simulink model "PVAndBatteryIntegratedPlantForBlackStart"  (R2025b)
settings: Solver=FixedStepAuto  StartTime=0.0  StopTime=tsim  FixedStep=1e-6  RelTol=1e-9  AbsTol=1e-7
InitFcn:
  | %% Black Start Sequence
  | t0 = 0; % Battery IBR initial time
  | t1 = 0.15; % PV IBR initial time
  | t2 = 0.5; % Two IBR sync time
  | t3 = 0.8; % Additional motor load connect
  | t4 = 1.1; % Grid reconnection
  | tsim = 1.5; % Total simulation time
  | 
  | %% initialize
  | Vdc = 400;
  | Vnom = 100;
  | Prated = 10000;
  | Qrated = 0;
  | Srated = sqrt(Prated^2+Qrated^2);
  | wnom = 2*pi*60;
  | fnom = 60;
  | Vminpu = 0.95;
  | 
  | kv = Vnom;
  | ki = 3*Vnom/Srated;
  | 
  | dwmax = 0.5*2*pi;
  | trisemax = 0.1;
  | 
  | C = 1/sqrt(2)/Vminpu^2/dwmax;
  | L = 1/C/wnom^2;
  | tau = C/kv/ki;
  | epsilon = sqrt(L/C);
  | ksy = 3/2/trisemax;
  | 
  | V_voc_1 = 0;
  | V_voc_2 = 0;
  | 
  | % filter
  | Rf = 0.05;
  | Lf = 500e-6;
  | % pwm
  | fsw = 10e3;
  | % simulation
  | Ts = 1e-6;
  | 
  | % load
  | Rl = 3*Vnom^2/Prated;
  | Rl1 = Rl;
  | Rl2 = 2*Rl;
  | Rl3 = 20*Rl;
  | % grid
  | Rg = 0.05;
  | Lg = 50e-6;
  | 
  | % DCDC converter
  | Kp_V = 1;
  | Ki_V = 0.02;
  | Imax = 110;
  | Kp_I = 0.0001;
  | Ki_I = 1;
  | Vcmax = 1;
undefined symbols (not defined in the file): alpha, C_voc, Diode_class, Half_BridgeConverter_class, L_voc, Ll, Mosfet_class, PWMGenerator_DC_DC__class, R_voc, Three_PhaseBreaker_class, Three_PhaseSource_class, Three_PhaseTransformer_2_class, Three_PhaseV_IMeasuremen_class
libraries: nesl_utility x69, ee_lib x49, fl_lib x36, mcbeeMathTransformLib x9, simulink x6, spsParallelRLCBranchLib x3, eePwmGeneratorTwoLevel x2, spsControlledCurrentSourceLib x2, elec_conv_HighZElecRef x2, slpidlib x2, spsSecondOrderFilterLib x1, spsCurrentMeasurementLib x1
(part 2 of 4)

== system PVAndBatteryIntegratedPlantForBlackStart/prim4 ==
  Current and Voltage Sensor (Three-Phase) : ee_lib/Sensors & Transducers/Current and Voltage Sensor (Three-Phase)  vMeasurementType=2  outputUnit=2  SRated=100000000 V*A  VRated=500000 V  I_specify=off  I_priority=None  I=[ 0 0 0 ] A  I_nominal_specify=off  I_nominal_value=1  I_nominal_unit=A  V_specify=off  V_priority=None  V=[ 0 0 0 ] V  V_nominal_specify=off  V_nominal_value=1  V_nominal_unit=V
      settings: InternalSimscapePortConfiguration="{\"Bottom\":[],\"Left\":[{\"id\":\"a1\",\"label\":\"a1\",\"type\":\"foundation.electrical.electrical\"},{\"id\":\"b1\",\"label\":\"b1\",\"type\":\"foundation.electrical.electrical\"},{\"id\":\"c1\",\"label\":\"c1\",\"type\":\"foundation.electrical.electrical\"}],\"Right\":[{\"id\":\"V_output\",\"label\":\"V\",\"type\":\"output\"},{\"id\":\"I_output\",\"label\":\"I\",\"type\":\"output\"},{\"id\":\"a2\",\"label\":\"a2\",\"type\":\"foundation.electrical.electrical\"},{\"id\":\"b2\",\"label\":\"b2\",\"type\":\"foundation.electrical.electrical\"},{\"id\":\"c2\",\"label\":\"c2\",\"type\":\"foundation.electrical.electrical\"}],\"Top\":[]}"
  Igain : Gain  Gain=Three_PhaseV_IMeasuremen_class('phase-to-ground','yes','off','off','off',100000000,500000).objParamMappingDerived.NewDerivedParam.IG
  PS-Simulink Converter : nesl_utility/PS-Simulink Converter  PhysicalDomain=network_engine_domain  SubClassName=ps_output  LeftPortType=input  RightPortType=output  PseudoPeriodic=off  Frequencies=[]  VectorFormat=1-D array  Unit=1  AffineConversion=off
  PS-Simulink Converter1 : nesl_utility/PS-Simulink Converter  PhysicalDomain=network_engine_domain  SubClassName=ps_output  LeftPortType=input  RightPortType=output  PseudoPeriodic=off  Frequencies=[]  VectorFormat=1-D array  Unit=1  AffineConversion=off
  Vgain : Gain  Gain=Three_PhaseV_IMeasuremen_class('phase-to-ground','yes','off','off','off',100000000,500000).objParamMappingDerived.NewDerivedParam.VG
  A : PMIOPort  Side=Left
  B : PMIOPort  Port=2  Side=Left
  C : PMIOPort  Port=3  Side=Left
  a : PMIOPort  Port=4  Side=Right
  b : PMIOPort  Port=5  Side=Right
  c : PMIOPort  Port=6  Side=Right
  Vabc : Outport  VectorParamsAs1DForOutWhenUnconnected=off
  Iabc : Outport  Port=2  VectorParamsAs1DForOutWhenUnconnected=off
  wires:
  Igain/1 -> Iabc/1
  Vgain/1 -> Vabc/1
  PS-Simulink Converter1/1 -> Igain/1
  PS-Simulink Converter/1 -> Vgain/1
  connections:
  Current and Voltage Sensor (Three-Phase)/RConn1 -- PS-Simulink Converter/LConn1
  Current and Voltage Sensor (Three-Phase)/RConn2 -- PS-Simulink Converter1/LConn1
  Current and Voltage Sensor (Three-Phase)/RConn5 -- c/RConn1
  Current and Voltage Sensor (Three-Phase)/RConn4 -- b/RConn1
  Current and Voltage Sensor (Three-Phase)/RConn3 -- a/RConn1
  Current and Voltage Sensor (Three-Phase)/LConn3 -- C/RConn1
  Current and Voltage Sensor (Three-Phase)/LConn1 -- A/RConn1
  Current and Voltage Sensor (Three-Phase)/LConn2 -- B/RConn1

== system PVAndBatteryIntegratedPlantForBlackStart/Battery Inverter/DC Voltage Source ==
  DC Voltage Source : fl_lib/Electrical/Electrical Sources/DC Voltage Source  v0=Vdc V
  - : PMIOPort  Side=Left
  + : PMIOPort  Port=2  Side=Right
  connections:
  DC Voltage Source/RConn1 -- -/RConn1
  DC Voltage Source/LConn1 -- +/RConn1

== system PVAndBatteryIntegratedPlantForBlackStart/Battery Inverter/Feedback ==
  In2 : Inport
  Enable : EnablePort
  Ifb : Outport
  wires:
  In2/1 -> Ifb/1

== system PVAndBatteryIntegratedPlantForBlackStart/Battery Inverter/Inverter ==
  g : Inport
  Constant : Constant  Value=0
  Demux : Demux  Outputs=6
  Half-Bridge Converter : Subsystem
  Half-Bridge Converter1 : Subsystem
      settings: OpenFcn=elec.conv.unmask(gcb);
  Half-Bridge Converter2 : Subsystem
      settings: OpenFcn=elec.conv.unmask(gcb);
  Mux : Mux  Inputs=2
  Mux1 : Mux  Inputs=2
  Mux2 : Mux  Inputs=2
  Vdc+ : PMIOPort  Side=Left
  Vdc- : PMIOPort  Port=2  Side=Left
  Va : PMIOPort  Port=3  Side=Right
  Vb : PMIOPort  Port=4  Side=Right
  Vc : PMIOPort  Port=5  Side=Right
  wires:
  g/1 -> Demux/1
  Constant/1 -> Half-Bridge Converter2/2(BL), Half-Bridge Converter1/2(BL), Half-Bridge Converter/2(BL)
  Demux/1 -> Mux/1
  Demux/2 -> Mux/2
  Demux/4 -> Mux1/2
  Demux/3 -> Mux1/1
  Demux/5 -> Mux2/1
  Demux/6 -> Mux2/2
  Mux/1 -> Half-Bridge Converter/1(" g ")
  Mux1/1 -> Half-Bridge Converter1/1(" g ")
  Mux2/1 -> Half-Bridge Converter2/1(" g ")
  connections:
  Half-Bridge Converter/RConn1 -- Half-Bridge Converter2/RConn1 -- Half-Bridge Converter1/RConn1 -- Vdc+/RConn1
  Vdc-/RConn1 -- Half-Bridge Converter2/RConn2 -- Half-Bridge Converter1/RConn2 -- Half-Bridge Converter/RConn2
  Half-Bridge Converter1/LConn1 -- Vb/RConn1
  Vc/RConn1 -- Half-Bridge Converter2/LConn1
  Va/RConn1 -- Half-Bridge Converter/LConn1

== system PVAndBatteryIntegratedPlantForBlackStart/Battery Inverter/L1 ==
  Three_PhaseSeriesRLCBran : ee_lib/Passive/RLC Assemblies/RLC (Three-Phase)  port_option=ee.enum.threePhasePort.expanded  component_structure=4  R=Rf Ohm  L=Lf H  C=Inf F  R_parasitic=1e-6 Ohm  G_parasitic=1e-6 1/Ohm  IL_specify=on  IL_priority=High  IL=[0, 0, 0] A  IL_nominal_specify=off  IL_nominal_value=1  IL_nominal_unit=A  VC_specify=on  VC_priority=High  VC=[0, 0, 0] V  VC_nominal_specify=off  VC_nominal_value=1  VC_nominal_unit=V
      settings: InternalSimscapePortConfiguration="{\"Bottom\":[],\"Left\":[{\"id\":\"a1\",\"label\":\"a1\",\"type\":\"foundation.electrical.electrical\"},{\"id\":\"b1\",\"label\":\"b1\",\"type\":\"foundation.electrical.electrical\"},{\"id\":\"c1\",\"label\":\"c1\",\"type\":\"foundation.electrical.electrical\"}],\"Right\":[{\"id\":\"a2\",\"label\":\"a2\",\"type\":\"foundation.electrical.electrical\"},{\"id\":\"b2\",\"label\":\"b2\",\"type\":\"foundation.electrical.electrical\"},{\"id\":\"c2\",\"label\":\"c2\",\"type\":\"foundation.electrical.electrical\"}],\"Top\":[]}"
  A : PMIOPort  Side=Left
  B : PMIOPort  Port=2  Side=Left
  C : PMIOPort  Port=3  Side=Left
  a : PMIOPort  Port=4  Side=Right
  b : PMIOPort  Port=5  Side=Right
  c : PMIOPort  Port=6  Side=Right
  connections:
  Three_PhaseSeriesRLCBran/RConn3 -- c/RConn1
  Three_PhaseSeriesRLCBran/RConn2 -- b/RConn1
  Three_PhaseSeriesRLCBran/RConn1 -- a/RConn1
  C/RConn1 -- Three_PhaseSeriesRLCBran/LConn3
  B/RConn1 -- Three_PhaseSeriesRLCBran/LConn2
  A/RConn1 -- Three_PhaseSeriesRLCBran/LConn1

== system PVAndBatteryIntegratedPlantForBlackStart/Battery Inverter/Three-Phase Breaker ==
  com : Inport
  Add : Sum
  Circuit Breaker : ee_lib/Switches & Breakers/Circuit Breaker (Three-Phase)  R_closed=0.001 Ohm  G_open=Three_PhaseBreaker_class('open',1000000,Inf,[0.0166666666666667 0.0833333333333333],'on').objParamMappingDerived.NewDerivedParam.G_open 1/Ohm  threshold=0.5 V  breaker_behavior=ee.enum.switches.breakerBehavior.zeroCrossingEnable
      settings: InternalSimscapePortConfiguration="{\"Bottom\":[],\"Left\":[{\"id\":\"vT\",\"label\":\"vT\",\"type\":\"input\"},{\"id\":\"a1\",\"label\":\"a1\",\"type\":\"foundation.electrical.electrical\"},{\"id\":\"b1\",\"label\":\"b1\",\"type\":\"foundation.electrical.electrical\"},{\"id\":\"c1\",\"label\":\"c1\",\"type\":\"foundation.electrical.electrical\"}],\"Right\":[{\"id\":\"a2\",\"label\":\"a2\",\"type\":\"foundation.electrical.electrical\"},{\"id\":\"b2\",\"label\":\"b2\",\"type\":\"foundation.electrical.electrical\"},{\"id\":\"c2\",\"label\":\"c2\",\"type\":\"foundation.electrical.electrical\"}],\"Top\":[]}"
  Data Type Conversion : DataTypeConversion  OutDataTypeStr=double  SaturateOnIntegerOverflow=off  RndMeth=Floor
  NOT : Logic  Operator=NOT  IconShape=distinctive  AllPortsSameDT=off  OutDataTypeStr=boolean
  Simulink-PS Converter : nesl_utility/Simulink-PS Converter  PhysicalDomain=network_engine_domain  SubClassName=ps_input  LeftPortType=input  RightPortType=output  PseudoPeriodic=off  Frequencies=[]  NoiseDistribution=none  NoiseParameters=[]  Unit=1  AffineConversion=off  FilteringAndDerivatives=provide  SimscapeFilterOrder=1  InputFilterTimeConstant=0.001  UdotUserProvided=0
  Step : Step  Time=1e-6  Before=Three_PhaseBreaker_class('open',1000000,Inf,[0.0166666666666667 0.0833333333333333],'on').objParamMappingDerived.NewDerivedParam.StepInitialValue  After=0  SampleTime=0
  A : PMIOPort  Side=Left
  B : PMIOPort  Port=2  Side=Left
  C : PMIOPort  Port=3  Side=Left
  a : PMIOPort  Port=4  Side=Right
  b : PMIOPort  Port=5  Side=Right
  c : PMIOPort  Port=6  Side=Right
  wires:
  com/1 -> Add/1
  Add/1 -> NOT/1
  Step/1 -> Add/2
  Data Type Conversion/1 -> Simulink-PS Converter/1
  NOT/1 -> Data Type Conversion/1
  connections:
  Circuit Breaker/LConn1 -- Simulink-PS Converter/RConn1
  c/RConn1 -- Circuit Breaker/RConn3
  b/RConn1 -- Circuit Breaker/RConn2
  a/RConn1 -- Circuit Breaker/RConn1
  Circuit Breaker/LConn4 -- C/RConn1
  Circuit Breaker/LConn3 -- B/RConn1
  Circuit Breaker/LConn2 -- A/RConn1

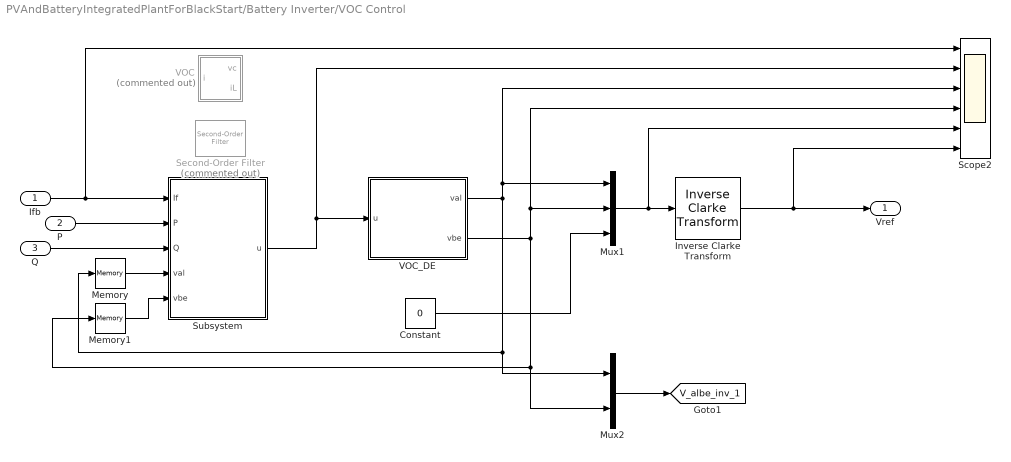
== system PVAndBatteryIntegratedPlantForBlackStart/Battery Inverter/VOC Control ==
  Ifb : Inport
  P : Inport  Port=2
  Q : Inport  Port=3
  Constant : Constant  Value=0
  Inverse Clarke Transform : mcbeeMathTransformLib/Inverse Clarke Transform  PowerInvariant=off  UseWithEmbedded=off  PhaseInput=Two inputs
      settings: LibrarySourceBlock=|
      | ee_sl_lib/Mathematical
      | Transforms/Inverse
      | Clarke Transform
  Memory : Memory
  Memory1 : Memory
  Mux1 : Mux  Inputs=3
  Mux2 : Mux  Inputs=2
  Scope2 : Scope  NumInputPorts=6
      settings: ActiveDisplayYMinimum=-957.42377  ActiveDisplayYMaximum=1099.35573
  Second-Order Filter : spsSecondOrderFilterLib/Second-Order Filter  Commented=on  FilterType=Lowpass  Fo=fnom*10  Zeta=0.707  Ts=0  Initialize=on  Vac_Init="[0,  0,  60]"  Vdc_Init=0  PlotResponse=off  FreqRange=[0, 500, 1]
      settings: LibrarySourceBlock=|
      | sps_lib/Control/Filters/Second-Order
      | Filter
  Subsystem : Subsystem
  VOC : Subsystem  Commented=on
  VOC_DE : Subsystem
  Vref : Outport
  tag scope: V_albe_inv_1=global
  wires:
  Memory1/1 -> Subsystem/5(vbe)
  Memory/1 -> Subsystem/4(val)
  Mux1/1 -> Scope2/5, Inverse Clarke Transform/1
  Ifb/1 -> Subsystem/1(If), Scope2/1
  Inverse Clarke Transform/1 -> Vref/1, Scope2/6
  VOC_DE/1(val) -> Mux2/1, Memory/1, Scope2/3, Mux1/1
  VOC_DE/2(vbe) -> Scope2/4, Mux1/2, Mux2/2, Memory1/1
  Constant/1 -> Mux1/3
  Subsystem/1(u) -> Scope2/2, VOC_DE/1(u)
  P/1 -> Subsystem/2(P)
  Q/1 -> Subsystem/3(Q)
  Mux2/1 -> [V_albe_inv_1]

== system PVAndBatteryIntegratedPlantForBlackStart/Battery Inverter/inv ==
  Current and Voltage Sensor (Three-Phase) : ee_lib/Sensors & Transducers/Current and Voltage Sensor (Three-Phase)  vMeasurementType=2  outputUnit=2  SRated=100000000 V*A  VRated=500000 V  I_specify=off  I_priority=None  I=[ 0 0 0 ] A  I_nominal_specify=off  I_nominal_value=1  I_nominal_unit=A  V_specify=off  V_priority=None  V=[ 0 0 0 ] V  V_nominal_specify=off  V_nominal_value=1  V_nominal_unit=V
      settings: InternalSimscapePortConfiguration="{\"Bottom\":[],\"Left\":[{\"id\":\"a1\",\"label\":\"a1\",\"type\":\"foundation.electrical.electrical\"},{\"id\":\"b1\",\"label\":\"b1\",\"type\":\"foundation.electrical.electrical\"},{\"id\":\"c1\",\"label\":\"c1\",\"type\":\"foundation.electrical.electrical\"}],\"Right\":[{\"id\":\"V_output\",\"label\":\"V\",\"type\":\"output\"},{\"id\":\"I_output\",\"label\":\"I\",\"type\":\"output\"},{\"id\":\"a2\",\"label\":\"a2\",\"type\":\"foundation.electrical.electrical\"},{\"id\":\"b2\",\"label\":\"b2\",\"type\":\"foundation.electrical.electrical\"},{\"id\":\"c2\",\"label\":\"c2\",\"type\":\"foundation.electrical.electrical\"}],\"Top\":[]}"
  Igain : Gain  Gain=Three_PhaseV_IMeasuremen_class('phase-to-ground','yes','off','off','off',100000000,500000).objParamMappingDerived.NewDerivedParam.IG
  PS-Simulink Converter : nesl_utility/PS-Simulink Converter  PhysicalDomain=network_engine_domain  SubClassName=ps_output  LeftPortType=input  RightPortType=output  PseudoPeriodic=off  Frequencies=[]  VectorFormat=1-D array  Unit=1  AffineConversion=off
  PS-Simulink Converter1 : nesl_utility/PS-Simulink Converter  PhysicalDomain=network_engine_domain  SubClassName=ps_output  LeftPortType=input  RightPortType=output  PseudoPeriodic=off  Frequencies=[]  VectorFormat=1-D array  Unit=1  AffineConversion=off
  Vgain : Gain  Gain=Three_PhaseV_IMeasuremen_class('phase-to-ground','yes','off','off','off',100000000,500000).objParamMappingDerived.NewDerivedParam.VG
  A : PMIOPort  Side=Left
  B : PMIOPort  Port=2  Side=Left
  C : PMIOPort  Port=3  Side=Left
  a : PMIOPort  Port=4  Side=Right
  b : PMIOPort  Port=5  Side=Right
  c : PMIOPort  Port=6  Side=Right
  Vabc : Outport  VectorParamsAs1DForOutWhenUnconnected=off
  Iabc : Outport  Port=2  VectorParamsAs1DForOutWhenUnconnected=off
  wires:
  Igain/1 -> Iabc/1
  Vgain/1 -> Vabc/1
  PS-Simulink Converter1/1 -> Igain/1
  PS-Simulink Converter/1 -> Vgain/1
  connections:
  Current and Voltage Sensor (Three-Phase)/RConn1 -- PS-Simulink Converter/LConn1
  Current and Voltage Sensor (Three-Phase)/RConn2 -- PS-Simulink Converter1/LConn1
  Current and Voltage Sensor (Three-Phase)/RConn5 -- c/RConn1
  Current and Voltage Sensor (Three-Phase)/RConn4 -- b/RConn1
  Current and Voltage Sensor (Three-Phase)/RConn3 -- a/RConn1
  Current and Voltage Sensor (Three-Phase)/LConn3 -- C/RConn1
  Current and Voltage Sensor (Three-Phase)/LConn1 -- A/RConn1
  Current and Voltage Sensor (Three-Phase)/LConn2 -- B/RConn1

== system PVAndBatteryIntegratedPlantForBlackStart/Battery Inverter/inv1 ==
  Current and Voltage Sensor (Three-Phase) : ee_lib/Sensors & Transducers/Current and Voltage Sensor (Three-Phase)  vMeasurementType=2  outputUnit=2  SRated=100000000 V*A  VRated=500000 V  I_specify=off  I_priority=None  I=[ 0 0 0 ] A  I_nominal_specify=off  I_nominal_value=1  I_nominal_unit=A  V_specify=off  V_priority=None  V=[ 0 0 0 ] V  V_nominal_specify=off  V_nominal_value=1  V_nominal_unit=V
      settings: InternalSimscapePortConfiguration="{\"Bottom\":[],\"Left\":[{\"id\":\"a1\",\"label\":\"a1\",\"type\":\"foundation.electrical.electrical\"},{\"id\":\"b1\",\"label\":\"b1\",\"type\":\"foundation.electrical.electrical\"},{\"id\":\"c1\",\"label\":\"c1\",\"type\":\"foundation.electrical.electrical\"}],\"Right\":[{\"id\":\"V_output\",\"label\":\"V\",\"type\":\"output\"},{\"id\":\"I_output\",\"label\":\"I\",\"type\":\"output\"},{\"id\":\"a2\",\"label\":\"a2\",\"type\":\"foundation.electrical.electrical\"},{\"id\":\"b2\",\"label\":\"b2\",\"type\":\"foundation.electrical.electrical\"},{\"id\":\"c2\",\"label\":\"c2\",\"type\":\"foundation.electrical.electrical\"}],\"Top\":[]}"
  Igain : Gain  Gain=Three_PhaseV_IMeasuremen_class('phase-to-ground','yes','off','off','off',100000000,500000).objParamMappingDerived.NewDerivedParam.IG
  PS-Simulink Converter : nesl_utility/PS-Simulink Converter  PhysicalDomain=network_engine_domain  SubClassName=ps_output  LeftPortType=input  RightPortType=output  PseudoPeriodic=off  Frequencies=[]  VectorFormat=1-D array  Unit=1  AffineConversion=off
  PS-Simulink Converter1 : nesl_utility/PS-Simulink Converter  PhysicalDomain=network_engine_domain  SubClassName=ps_output  LeftPortType=input  RightPortType=output  PseudoPeriodic=off  Frequencies=[]  VectorFormat=1-D array  Unit=1  AffineConversion=off
  Vgain : Gain  Gain=Three_PhaseV_IMeasuremen_class('phase-to-ground','yes','off','off','off',100000000,500000).objParamMappingDerived.NewDerivedParam.VG
  A : PMIOPort  Side=Left
  B : PMIOPort  Port=2  Side=Left
  C : PMIOPort  Port=3  Side=Left
  a : PMIOPort  Port=4  Side=Right
  b : PMIOPort  Port=5  Side=Right
  c : PMIOPort  Port=6  Side=Right
  Vabc : Outport  VectorParamsAs1DForOutWhenUnconnected=off
  Iabc : Outport  Port=2  VectorParamsAs1DForOutWhenUnconnected=off
  wires:
  Igain/1 -> Iabc/1
  Vgain/1 -> Vabc/1
  PS-Simulink Converter1/1 -> Igain/1
  PS-Simulink Converter/1 -> Vgain/1
  connections:
  Current and Voltage Sensor (Three-Phase)/RConn1 -- PS-Simulink Converter/LConn1
  Current and Voltage Sensor (Three-Phase)/RConn2 -- PS-Simulink Converter1/LConn1
  Current and Voltage Sensor (Three-Phase)/RConn5 -- c/RConn1
  Current and Voltage Sensor (Three-Phase)/RConn4 -- b/RConn1
  Current and Voltage Sensor (Three-Phase)/RConn3 -- a/RConn1
  Current and Voltage Sensor (Three-Phase)/LConn3 -- C/RConn1
  Current and Voltage Sensor (Three-Phase)/LConn1 -- A/RConn1
  Current and Voltage Sensor (Three-Phase)/LConn2 -- B/RConn1

== system PVAndBatteryIntegratedPlantForBlackStart/Linear Load 2/Three-Phase Series RLC Branch1 ==
  Three_PhaseSeriesRLCBran : ee_lib/Passive/RLC Assemblies/RLC (Three-Phase)  port_option=ee.enum.threePhasePort.expanded  component_structure=1  R=Rl2 Ohm  L=Ll H  C=1e-06 F  R_parasitic=1e-6 Ohm  G_parasitic=1e-6 1/Ohm  IL_specify=on  IL_priority=High  IL=[0, 0, 0] A  IL_nominal_specify=off  IL_nominal_value=1  IL_nominal_unit=A  VC_specify=on  VC_priority=High  VC=[0, 0, 0] V  VC_nominal_specify=off  VC_nominal_value=1  VC_nominal_unit=V
      settings: InternalSimscapePortConfiguration="{\"Bottom\":[],\"Left\":[{\"id\":\"a1\",\"label\":\"a1\",\"type\":\"foundation.electrical.electrical\"},{\"id\":\"b1\",\"label\":\"b1\",\"type\":\"foundation.electrical.electrical\"},{\"id\":\"c1\",\"label\":\"c1\",\"type\":\"foundation.electrical.electrical\"}],\"Right\":[{\"id\":\"a2\",\"label\":\"a2\",\"type\":\"foundation.electrical.electrical\"},{\"id\":\"b2\",\"label\":\"b2\",\"type\":\"foundation.electrical.electrical\"},{\"id\":\"c2\",\"label\":\"c2\",\"type\":\"foundation.electrical.electrical\"}],\"Top\":[]}"
  A : PMIOPort  Side=Left
  B : PMIOPort  Port=2  Side=Left
  C : PMIOPort  Port=3  Side=Left
  a : PMIOPort  Port=4  Side=Right
  b : PMIOPort  Port=5  Side=Right
  c : PMIOPort  Port=6  Side=Right
  connections:
  Three_PhaseSeriesRLCBran/RConn3 -- c/RConn1
  Three_PhaseSeriesRLCBran/RConn2 -- b/RConn1
  Three_PhaseSeriesRLCBran/RConn1 -- a/RConn1
  C/RConn1 -- Three_PhaseSeriesRLCBran/LConn3
  B/RConn1 -- Three_PhaseSeriesRLCBran/LConn2
  A/RConn1 -- Three_PhaseSeriesRLCBran/LConn1

== system PVAndBatteryIntegratedPlantForBlackStart/Linear load 1/Three-Phase Series RLC Branch ==
  Three_PhaseSeriesRLCBran : ee_lib/Passive/RLC Assemblies/RLC (Three-Phase)  port_option=ee.enum.threePhasePort.expanded  component_structure=1  R=Rl1 Ohm  L=Ll H  C=1e-06 F  R_parasitic=1e-6 Ohm  G_parasitic=1e-6 1/Ohm  IL_specify=on  IL_priority=High  IL=[0, 0, 0] A  IL_nominal_specify=off  IL_nominal_value=1  IL_nominal_unit=A  VC_specify=on  VC_priority=High  VC=[0, 0, 0] V  VC_nominal_specify=off  VC_nominal_value=1  VC_nominal_unit=V
      settings: InternalSimscapePortConfiguration="{\"Bottom\":[],\"Left\":[{\"id\":\"a1\",\"label\":\"a1\",\"type\":\"foundation.electrical.electrical\"},{\"id\":\"b1\",\"label\":\"b1\",\"type\":\"foundation.electrical.electrical\"},{\"id\":\"c1\",\"label\":\"c1\",\"type\":\"foundation.electrical.electrical\"}],\"Right\":[{\"id\":\"a2\",\"label\":\"a2\",\"type\":\"foundation.electrical.electrical\"},{\"id\":\"b2\",\"label\":\"b2\",\"type\":\"foundation.electrical.electrical\"},{\"id\":\"c2\",\"label\":\"c2\",\"type\":\"foundation.electrical.electrical\"}],\"Top\":[]}"
  A : PMIOPort  Side=Left
  B : PMIOPort  Port=2  Side=Left
  C : PMIOPort  Port=3  Side=Left
  a : PMIOPort  Port=4  Side=Right
  b : PMIOPort  Port=5  Side=Right
  c : PMIOPort  Port=6  Side=Right
  connections:
  Three_PhaseSeriesRLCBran/RConn3 -- c/RConn1
  Three_PhaseSeriesRLCBran/RConn2 -- b/RConn1
  Three_PhaseSeriesRLCBran/RConn1 -- a/RConn1
  C/RConn1 -- Three_PhaseSeriesRLCBran/LConn3
  B/RConn1 -- Three_PhaseSeriesRLCBran/LConn2
  A/RConn1 -- Three_PhaseSeriesRLCBran/LConn1

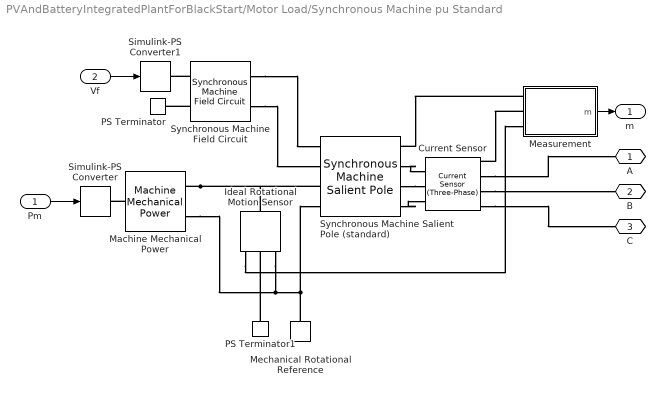
== system PVAndBatteryIntegratedPlantForBlackStart/Motor Load/Synchronous Machine pu Standard ==
  Pm : Inport
  Vf : Inport  Port=2
  Current Sensor : ee_lib/Sensors & Transducers/Current Sensor (Three-Phase)
      settings: InternalSimscapePortConfiguration="{\"Bottom\":[],\"Left\":[{\"id\":\"a1\",\"label\":\"a1\",\"type\":\"foundation.electrical.electrical\"},{\"id\":\"b1\",\"label\":\"b1\",\"type\":\"foundation.electrical.electrical\"},{\"id\":\"c1\",\"label\":\"c1\",\"type\":\"foundation.electrical.electrical\"}],\"Right\":[{\"id\":\"I_output\",\"label\":\"I\",\"type\":\"output\"},{\"id\":\"a2\",\"label\":\"a2\",\"type\":\"foundation.electrical.electrical\"},{\"id\":\"b2\",\"label\":\"b2\",\"type\":\"foundation.electrical.electrical\"},{\"id\":\"c2\",\"label\":\"c2\",\"type\":\"foundation.electrical.electrical\"}],\"Top\":[]}"
  Ideal Rotational Motion Sensor : fl_lib/Mechanical/Mechanical Sensors/Ideal Rotational Motion Sensor  reference=foundation.enum.MeasurementReference.difference  acceleration_port=false  velocity_port=true  position_port=true  wrap_angle=simscape.enum.onoff.on  offset=SynchronousMachinePuStan_class('Mechanical power Pm',[6000 122.5 60],[0.1028 0.02056 2],20,[0 0 0 0 0 0 0 0 1],[0.6404 0.7127 0.8441 0.9214 0.9956 1.082 1.19 1.316 1.457;0.7 0.7698 0.8872 0.9466 0.9969 1.046 1.1 1.151 1.201],'on','Salient-pole','Short-circuit','Short-circuit',[1.81 0.3 0.23 1.76 0.65 0.25 0.15],[2.24 0.17 0.12 1.02 0.13 0.08],[4.4849 0.0681 0.1],[8 0.03 1 0.07],[4.49 0.0681 0.0513],[8 0.03 0.3371 0.0295],[1.01 0.053 0.1],[1.3201 0.023 1 0.07],[0.012 0.003 0.003],[1.3201 0.0231 0.3371 0.0295]).objParamMappingDerived.NewDerivedParam.thm0 deg
  Machine Mechanical Power : ee_lib/Electromechanical/Mechanical/Machine Mechanical Power  power_sign=-1  SRated=6000 V*A  FRated=60 Hz  nPolePairs=2  inputUnit=ee.enum.unit.pu  torque_factor=2  inertia_option=2  J=27548 kg*m^2  H=0.1028 s*W/V/A  damper_option=2  D=39.0509 N*m/(rad/s)  pu_D=0.02056  initialization_option=2  fMechanical0=60 Hz  fElectrical0=SynchronousMachinePuStan_class('Mechanical power Pm',[6000 122.5 60],[0.1028 0.02056 2],20,[0 0 0 0 0 0 0 0 1],[0.6404 0.7127 0.8441 0.9214 0.9956 1.082 1.19 1.316 1.457;0.7 0.7698 0.8872 0.9466 0.9969 1.046 1.1 1.151 1.201],'on','Salient-pole','Short-circuit','Short-circuit',[1.81 0.3 0.23 1.76 0.65 0.25 0.15],[2.24 0.17 0.12 1.02 0.13 0.08],[4.4849 0.0681 0.1],[8 0.03 1 0.07],[4.49 0.0681 0.0513],[8 0.03 0.3371 0.0295],[1.01 0.053 0.1],[1.3201 0.023 1 0.07],[0.012 0.003 0.003],[1.3201 0.0231 0.3371 0.0295]).objParamMappingDerived.NewDerivedParam.fElectrical0 Hz
      settings: InternalSimscapePortConfiguration="{\"Bottom\":[],\"Left\":[{\"id\":\"Pm_pu\",\"label\":\"pu\",\"type\":\"input\"}],\"Right\":[{\"id\":\"R\",\"label\":\"R\",\"type\":\"foundation.mechanical.rotational.rotational\"},{\"id\":\"C\",\"label\":\"C\",\"type\":\"foundation.mechanical.rotational.rotational\"}],\"Top\":[]}"
  Measurement : Subsystem
  Mechanical Rotational Reference : fl_lib/Mechanical/Rotational Elements/Mechanical Rotational Reference
  PS Terminator : fl_lib/Physical Signals/Sinks/PS Terminator
  PS Terminator1 : fl_lib/Physical Signals/Sinks/PS Terminator
  Simulink-PS Converter : nesl_utility/Simulink-PS Converter  PhysicalDomain=network_engine_domain  SubClassName=ps_input  LeftPortType=input  RightPortType=output  PseudoPeriodic=off  Frequencies=[]  NoiseDistribution=none  NoiseParameters=[]  Unit=1  AffineConversion=off  FilteringAndDerivatives=provide  SimscapeFilterOrder=1  InputFilterTimeConstant=0.001  UdotUserProvided=0
  Simulink-PS Converter1 : nesl_utility/Simulink-PS Converter  PhysicalDomain=network_engine_domain  SubClassName=ps_input  LeftPortType=input  RightPortType=output  PseudoPeriodic=off  Frequencies=[]  NoiseDistribution=none  NoiseParameters=[]  Unit=1  AffineConversion=off  FilteringAndDerivatives=provide  SimscapeFilterOrder=1  InputFilterTimeConstant=0.001  UdotUserProvided=0
  Synchronous Machine Field Circuit : ee_lib/Electromechanical/Synchronous/Synchronous Machine Field Circuit  unit_option=ee.enum.unit.pu  SRated=6000 V*A  FRated=60 Hz  fieldCircuitParameterization_option=ee.enum.sm.fieldparameterization.current  baseEfd=92.95 V  baseIfd=SynchronousMachinePuStan_class('Mechanical power Pm',[6000 122.5 60],[0.1028 0.02056 2],20,[0 0 0 0 0 0 0 0 1],[0.6404 0.7127 0.8441 0.9214 0.9956 1.082 1.19 1.316 1.457;0.7 0.7698 0.8872 0.9466 0.9969 1.046 1.1 1.151 1.201],'on','Salient-pole','Short-circuit','Short-circuit',[1.81 0.3 0.23 1.76 0.65 0.25 0.15],[2.24 0.17 0.12 1.02 0.13 0.08],[4.4849 0.0681 0.1],[8 0.03 1 0.07],[4.49 0.0681 0.0513],[8 0.03 0.3371 0.0295],[1.01 0.053 0.1],[1.3201 0.023 1 0.07],[0.012 0.003 0.003],[1.3201 0.0231 0.3371 0.0295]).objParamMappingDerived.NewDerivedParam.baseIfd A  parameterization_option=ee.enum.sm.parameterization.standard  Ladu=1.66  Rfd=0.0006  Xl=0.08  Xd=2.24  Xdd=0.17  Xddd=0.12  d_option=2  Td0d=8 s  Tdd=0.012 s  Td0dd=0.05 s  Tddd=0.003 s
      settings: InternalSimscapePortConfiguration="{\"Bottom\":[],\"Left\":[{\"id\":\"Efd_pu\",\"label\":\"Efd_pu\",\"type\":\"input\"},{\"id\":\"Ifd_pu\",\"label\":\"Ifd_pu\",\"type\":\"output\"}],\"Right\":[{\"id\":\"fd_p\",\"label\":\"fd+\",\"type\":\"foundation.electrical.electrical\"},{\"id\":\"fd_n\",\"label\":\"fd-\",\"type\":\"foundation.electrical.electrical\"}],\"Top\":[]}"
  Synchronous Machine Salient Pole (standard) : ee_lib/Electromechanical/Synchronous/Synchronous Machine Salient Pole  port_option=ee.enum.threePhasePort.expanded  SRated=6000 V*A  VRated=122.5 V  FRated=60 Hz  nPolePairs=2  param_option=ee.enum.sm.parameterization.standard  fieldCircuitParameterization_option=ee.enum.sm.fieldparameterization.current  baseEfd=216.54 V  baseIfd=SynchronousMachinePuStan_class('Mechanical power Pm',[6000 122.5 60],[0.1028 0.02056 2],20,[0 0 0 0 0 0 0 0 1],[0.6404 0.7127 0.8441 0.9214 0.9956 1.082 1.19 1.316 1.457;0.7 0.7698 0.8872 0.9466 0.9969 1.046 1.1 1.151 1.201],'on','Salient-pole','Short-circuit','Short-circuit',[1.81 0.3 0.23 1.76 0.65 0.25 0.15],[2.24 0.17 0.12 1.02 0.13 0.08],[4.4849 0.0681 0.1],[8 0.03 1 0.07],[4.49 0.0681 0.0513],[8 0.03 0.3371 0.0295],[1.01 0.053 0.1],[1.3201 0.023 1 0.07],[0.012 0.003 0.003],[1.3201 0.0231 0.3371 0.0295]).objParamMappingDerived.NewDerivedParam.baseIfd A  zero_sequence=ee.enum.park.zerosequence.exclude  axes_param=ee.enum.rotorangle.qaxis  Ladu=0.9  Laqu=0.55  L0=0.15  Ll=0.15  Ra=0.037875  Lfd=0.2571  Rfd=0.0006  L1d=0.2  R1d=0.0354  L1q=0.2567  R1q=0.0428  Xl=0.08  Xd=2.24  Xq=1.02  X0=0.08  Xdd=0.17  Xddd=0.12  Xqdd=0.13  d_option=2  Td0d=8 s  Tdd=0.012 s  Td0dd=0.05 s  Tddd=0.003 s  q_option=2  Tq0dd=0.05 s  Tqdd=0.003 s  saturation_option=1  saturation_ifd=SynchronousMachinePuStan_class('Mechanical power Pm',[6000 122.5 60],[0.1028 0.02056 2],20,[0 0 0 0 0 0 0 0 1],[0.6404 0.7127 0.8441 0.9214 0.9956 1.082 1.19 1.316 1.457;0.7 0.7698 0.8872 0.9466 0.9969 1.046 1.1 1.151 1.201],'on','Salient-pole','Short-circuit','Short-circuit',[1.81 0.3 0.23 1.76 0.65 0.25 0.15],[2.24 0.17 0.12 1.02 0.13 0.08],[4.4849 0.0681 0.1],[8 0.03 1 0.07],[4.49 0.0681 0.0513],[8 0.03 0.3371 0.0295],[1.01 0.053 0.1],[1.3201 0.023 1 0.07],[0.012 0.003 0.003],[1.3201 0.0231 0.3371 0.0295]).objParamMappingDerived.NewDerivedParam.saturation_ifd  saturation_Vag=SynchronousMachinePuStan_class('Mechanical power Pm',[6000 122.5 60],[0.1028 0.02056 2],20,[0 0 0 0 0 0 0 0 1],[0.6404 0.7127 0.8441 0.9214 0.9956 1.082 1.19 1.316 1.457;0.7 0.7698 0.8872 0.9466 0.9969 1.046 1.1 1.151 1.201],'on','Salient-pole','Short-circuit','Short-circuit',[1.81 0.3 0.23 1.76 0.65 0.25 0.15],[2.24 0.17 0.12 1.02 0.13 0.08],[4.4849 0.0681 0.1],[8 0.03 1 0.07],[4.49 0.0681 0.0513],[8 0.03 0.3371 0.0295],[1.01 0.053 0.1],[1.3201 0.023 1 0.07],[0.012 0.003 0.003],[1.3201 0.0231 0.3371 0.0295]).objParamMappingDerived.NewDerivedParam.saturation_Vag  initialization_option=ee.enum.sm.initialization.mechanical  source_type=ee.enum.sm.load_flow_source_type.Swing  Vmag0=24e3 V  Vang0=0 deg  Pt0=270e6 V*A  Qt0=0 V*A  minimum_pu=0.95  phase_search_range=[-30, 30] deg  gmin=1e-6 S  connection_option=ee.enum.Connection.wye  num_q_dampers=1  rotor_offset=-pi / 2 rad  pu_psid_specify=on  pu_psid_priority=High  pu_psid=SynchronousMachinePuStan_class('Mechanical power Pm',[6000 122.5 60],[0.1028 0.02056 2],20,[0 0 0 0 0 0 0 0 1],[0.6404 0.7127 0.8441 0.9214 0.9956 1.082 1.19 1.316 1.457;0.7 0.7698 0.8872 0.9466 0.9969 1.046 1.1 1.151 1.201],'on','Salient-pole','Short-circuit','Short-circuit',[1.81 0.3 0.23 1.76 0.65 0.25 0.15],[2.24 0.17 0.12 1.02 0.13 0.08],[4.4849 0.0681 0.1],[8 0.03 1 0.07],[4.49 0.0681 0.0513],[8 0.03 0.3371 0.0295],[1.01 0.053 0.1],[1.3201 0.023 1 0.07],[0.012 0.003 0.003],[1.3201 0.0231 0.3371 0.0295]).objParamMappingDerived.NewDerivedParam.pu_psid0  pu_psid_nominal_specify=off  pu_psid_nominal_value=1  pu_psid_nominal_unit=1  pu_psiq_specify=on  pu_psiq_priority=High  pu_psiq=SynchronousMachinePuStan_class('Mechanical power Pm',[6000 122.5 60],[0.1028 0.02056 2],20,[0 0 0 0 0 0 0 0 1],[0.6404 0.7127 0.8441 0.9214 0.9956 1.082 1.19 1.316 1.457;0.7 0.7698 0.8872 0.9466 0.9969 1.046 1.1 1.151 1.201],'on','Salient-pole','Short-circuit','Short-circuit',[1.81 0.3 0.23 1.76 0.65 0.25 0.15],[2.24 0.17 0.12 1.02 0.13 0.08],[4.4849 0.0681 0.1],[8 0.03 1 0.07],[4.49 0.0681 0.0513],[8 0.03 0.3371 0.0295],[1.01 0.053 0.1],[1.3201 0.023 1 0.07],[0.012 0.003 0.003],[1.3201 0.0231 0.3371 0.0295]).objParamMappingDerived.NewDerivedParam.pu_psiq0  pu_psiq_nominal_specify=off  pu_psiq_nominal_value=1  pu_psiq_nominal_unit=1  pu_psifd_specify=on  pu_psifd_priority=High  pu_psifd=SynchronousMachinePuStan_class('Mechanical power Pm',[6000 122.5 60],[0.1028 0.02056 2],20,[0 0 0 0 0 0 0 0 1],[0.6404 0.7127 0.8441 0.9214 0.9956 1.082 1.19 1.316 1.457;0.7 0.7698 0.8872 0.9466 0.9969 1.046 1.1 1.151 1.201],'on','Salient-pole','Short-circuit','Short-circuit',[1.81 0.3 0.23 1.76 0.65 0.25 0.15],[2.24 0.17 0.12 1.02 0.13 0.08],[4.4849 0.0681 0.1],[8 0.03 1 0.07],[4.49 0.0681 0.0513],[8 0.03 0.3371 0.0295],[1.01 0.053 0.1],[1.3201 0.023 1 0.07],[0.012 0.003 0.003],[1.3201 0.0231 0.3371 0.0295]).objParamMappingDerived.NewDerivedParam.pu_psifd0  pu_psifd_nominal_specify=off  pu_psifd_nominal_value=1  pu_psifd_nominal_unit=1  pu_psi1d_specify=on  pu_psi1d_priority=High  pu_psi1d=SynchronousMachinePuStan_class('Mechanical power Pm',[6000 122.5 60],[0.1028 0.02056 2],20,[0 0 0 0 0 0 0 0 1],[0.6404 0.7127 0.8441 0.9214 0.9956 1.082 1.19 1.316 1.457;0.7 0.7698 0.8872 0.9466 0.9969 1.046 1.1 1.151 1.201],'on','Salient-pole','Short-circuit','Short-circuit',[1.81 0.3 0.23 1.76 0.65 0.25 0.15],[2.24 0.17 0.12 1.02 0.13 0.08],[4.4849 0.0681 0.1],[8 0.03 1 0.07],[4.49 0.0681 0.0513],[8 0.03 0.3371 0.0295],[1.01 0.053 0.1],[1.3201 0.023 1 0.07],[0.012 0.003 0.003],[1.3201 0.0231 0.3371 0.0295]).objParamMappingDerived.NewDerivedParam.pu_psi1d0  pu_psi1d_nominal_specify=off  pu_psi1d_nominal_value=1  pu_psi1d_nominal_unit=1  pu_psi1q_specify=on  pu_psi1q_priority=High  pu_psi1q=SynchronousMachinePuStan_class('Mechanical power Pm',[6000 122.5 60],[0.1028 0.02056 2],20,[0 0 0 0 0 0 0 0 1],[0.6404 0.7127 0.8441 0.9214 0.9956 1.082 1.19 1.316 1.457;0.7 0.7698 0.8872 0.9466 0.9969 1.046 1.1 1.151 1.201],'on','Salient-pole','Short-circuit','Short-circuit',[1.81 0.3 0.23 1.76 0.65 0.25 0.15],[2.24 0.17 0.12 1.02 0.13 0.08],[4.4849 0.0681 0.1],[8 0.03 1 0.07],[4.49 0.0681 0.0513],[8 0.03 0.3371 0.0295],[1.01 0.053 0.1],[1.3201 0.023 1 0.07],[0.012 0.003 0.003],[1.3201 0.0231 0.3371 0.0295]).objParamMappingDerived.NewDerivedParam.pu_psi1q0  pu_psi1q_nominal_specify=off  pu_psi1q_nominal_value=1  pu_psi1q_nominal_unit=1  angular_position_diff_specify=on  angular_position_diff_priority=High  angular_position_diff=SynchronousMachinePuStan_class('Mechanical power Pm',[6000 122.5 60],[0.1028 0.02056 2],20,[0 0 0 0 0 0 0 0 1],[0.6404 0.7127 0.8441 0.9214 0.9956 1.082 1.19 1.316 1.457;0.7 0.7698 0.8872 0.9466 0.9969 1.046 1.1 1.151 1.201],'on','Salient-pole','Short-circuit','Short-circuit',[1.81 0.3 0.23 1.76 0.65 0.25 0.15],[2.24 0.17 0.12 1.02 0.13 0.08],[4.4849 0.0681 0.1],[8 0.03 1 0.07],[4.49 0.0681 0.0513],[8 0.03 0.3371 0.0295],[1.01 0.053 0.1],[1.3201 0.023 1 0.07],[0.012 0.003 0.003],[1.3201 0.0231 0.3371 0.0295]).objParamMappingDerived.NewDerivedParam.thm0 deg  angular_position_diff_nominal_specify=off  angular_position_diff_nominal_value=1  angular_position_diff_nominal_unit=deg  Tmeas=298.15 K  alpha=3.93e-3 1/K  stator_thermal_mass=100 J/K  rotor_thermal_mass=200 J/K  temperatureA_specify=off  temperatureA_priority=High  temperatureA=25 degC  temperatureA_nominal_specify=off  temperatureA_nominal_value=1  temperatureA_nominal_unit=degC  temperatureB_specify=off  temperatureB_priority=High  temperatureB=25 degC  temperatureB_nominal_specify=off  temperatureB_nominal_value=1  temperatureB_nominal_unit=degC  temperatureC_specify=off  temperatureC_priority=High  temperatureC=25 degC  temperatureC_nominal_specify=off  temperatureC_nominal_value=1  temperatureC_nominal_unit=degC  temperatureR_specify=off  temperatureR_priority=High  temperatureR=25 degC  temperatureR_nominal_specify=off  temperatureR_nominal_value=1  temperatureR_nominal_unit=degC
      settings: InternalSimscapePortConfiguration="{\"Bottom\":[],\"Left\":[{\"id\":\"fd_p\",\"label\":\"fd+\",\"type\":\"foundation.electrical.electrical\"},{\"id\":\"fd_n\",\"label\":\"fd-\",\"type\":\"foundation.electrical.electrical\"},{\"id\":\"R\",\"label\":\"R\",\"type\":\"foundation.mechanical.rotational.rotational\"},{\"id\":\"C\",\"label\":\"C\",\"type\":\"foundation.mechanical.rotational.rotational\"}],\"Right\":[{\"id\":\"pu_output\",\"label\":\"pu\",\"type\":\"output\"},{\"id\":\"a\",\"label\":\"a\",\"type\":\"foundation.electrical.electrical\"},{\"id\":\"b\",\"label\":\"b\",\"type\":\"foundation.electrical.electrical\"},{\"id\":\"c\",\"label\":\"c\",\"type\":\"foundation.electrical.electrical\"}],\"Top\":[]}"
  A : PMIOPort  Side=Right
  B : PMIOPort  Port=2  Side=Right
  C : PMIOPort  Port=3  Side=Right
  m : Outport  VectorParamsAs1DForOutWhenUnconnected=off
  wires:
  Pm/1 -> Simulink-PS Converter/1
  Vf/1 -> Simulink-PS Converter1/1
  Measurement/1(m) -> m/1
  connections:
  Synchronous Machine Salient Pole (standard)/RConn2 -- Current Sensor/LConn1
  Ideal Rotational Motion Sensor/RConn3 -- Measurement/LConn3
  PS Terminator1/LConn1 -- Ideal Rotational Motion Sensor/RConn2
  Synchronous Machine Field Circuit/LConn2 -- PS Terminator/LConn1
  Synchronous Machine Field Circuit/LConn1 -- Simulink-PS Converter1/RConn1
  Synchronous Machine Field Circuit/RConn1 -- Synchronous Machine Salient Pole (standard)/LConn1
  Synchronous Machine Field Circuit/RConn2 -- Synchronous Machine Salient Pole (standard)/LConn2
  Machine Mechanical Power/RConn1 -- Ideal Rotational Motion Sensor/LConn1 -- Synchronous Machine Salient Pole (standard)/LConn3
  Machine Mechanical Power/RConn2 -- Ideal Rotational Motion Sensor/RConn1 -- Synchronous Machine Salient Pole (standard)/LConn4 -- Mechanical Rotational Reference/LConn1
  Machine Mechanical Power/LConn1 -- Simulink-PS Converter/RConn1
  Synchronous Machine Salient Pole (standard)/RConn3 -- Current Sensor/LConn2
  Synchronous Machine Salient Pole (standard)/RConn4 -- Current Sensor/LConn3
  Current Sensor/RConn2 -- A/RConn1
  Current Sensor/RConn3 -- B/RConn1
  Current Sensor/RConn4 -- C/RConn1
  Measurement/LConn1 -- Synchronous Machine Salient Pole (standard)/RConn1
  Measurement/LConn2 -- Current Sensor/RConn1

== system PVAndBatteryIntegratedPlantForBlackStart/Motor Load/Three-Phase Series RLC Branch3 ==
  Three_PhaseSeriesRLCBran : ee_lib/Passive/RLC Assemblies/RLC (Three-Phase)  port_option=ee.enum.threePhasePort.expanded  component_structure=1  R=Rl3 Ohm  L=Ll H  C=1e-06 F  R_parasitic=1e-6 Ohm  G_parasitic=1e-6 1/Ohm  IL_specify=on  IL_priority=High  IL=[0, 0, 0] A  IL_nominal_specify=off  IL_nominal_value=1  IL_nominal_unit=A  VC_specify=on  VC_priority=High  VC=[0, 0, 0] V  VC_nominal_specify=off  VC_nominal_value=1  VC_nominal_unit=V
      settings: InternalSimscapePortConfiguration="{\"Bottom\":[],\"Left\":[{\"id\":\"a1\",\"label\":\"a1\",\"type\":\"foundation.electrical.electrical\"},{\"id\":\"b1\",\"label\":\"b1\",\"type\":\"foundation.electrical.electrical\"},{\"id\":\"c1\",\"label\":\"c1\",\"type\":\"foundation.electrical.electrical\"}],\"Right\":[{\"id\":\"a2\",\"label\":\"a2\",\"type\":\"foundation.electrical.electrical\"},{\"id\":\"b2\",\"label\":\"b2\",\"type\":\"foundation.electrical.electrical\"},{\"id\":\"c2\",\"label\":\"c2\",\"type\":\"foundation.electrical.electrical\"}],\"Top\":[]}"
  A : PMIOPort  Side=Left
  B : PMIOPort  Port=2  Side=Left
  C : PMIOPort  Port=3  Side=Left
  a : PMIOPort  Port=4  Side=Right
  b : PMIOPort  Port=5  Side=Right
  c : PMIOPort  Port=6  Side=Right
  connections:
  Three_PhaseSeriesRLCBran/RConn3 -- c/RConn1
  Three_PhaseSeriesRLCBran/RConn2 -- b/RConn1
  Three_PhaseSeriesRLCBran/RConn1 -- a/RConn1
  C/RConn1 -- Three_PhaseSeriesRLCBran/LConn3
  B/RConn1 -- Three_PhaseSeriesRLCBran/LConn2
  A/RConn1 -- Three_PhaseSeriesRLCBran/LConn1

== system PVAndBatteryIntegratedPlantForBlackStart/PV Inverter /Current Measurement ==
  Current Sensor : fl_lib/Electrical/Electrical Sensors/Current Sensor
  PS-Simulink Converter : nesl_utility/PS-Simulink Converter  PhysicalDomain=network_engine_domain  SubClassName=ps_output  LeftPortType=input  RightPortType=output  PseudoPeriodic=off  Frequencies=[]  VectorFormat=1-D array  Unit=A  AffineConversion=off
  + : PMIOPort  Side=Left
  - : PMIOPort  Port=2  Side=Right
  i : Outport  VectorParamsAs1DForOutWhenUnconnected=off
  wires:
  PS-Simulink Converter/1 -> i/1
  connections:
  +/RConn1 -- Current Sensor/LConn1
  -/RConn1 -- Current Sensor/RConn2
  PS-Simulink Converter/LConn1 -- Current Sensor/RConn1

== system PVAndBatteryIntegratedPlantForBlackStart/PV Inverter /Diode ==
  Diode : fl_lib/Electrical/Electrical Elements/Diode  Vf=Diode_class(0.001,500,2.5e-07,0.8).objParamMappingDerived.NewDerivedParam.Vf V  Ron=Diode_class(0.001,500,2.5e-07,0.8).objParamMappingDerived.NewDerivedParam.Ron Ohm  Goff=Diode_class(0.001,500,2.5e-07,0.8).objParamMappingDerived.NewDerivedParam.Goff 1/Ohm  i_specify=off  i_priority=None  i=0 A  i_nominal_specify=off  i_nominal_value=1  i_nominal_unit=A  v_specify=off  v_priority=None  v=0 V  v_nominal_specify=off  v_nominal_value=1  v_nominal_unit=V
  a : PMIOPort  Side=Left
  k : PMIOPort  Port=2  Side=Right
  connections:
  k/RConn1 -- Diode/RConn1
  a/RConn1 -- Diode/LConn1

== system PVAndBatteryIntegratedPlantForBlackStart/PV Inverter /Feedback ==
  In2 : Inport
  Enable : EnablePort
  Ifb : Outport
  wires:
  In2/1 -> Ifb/1

== system PVAndBatteryIntegratedPlantForBlackStart/PV Inverter /Inverter ==
  g : Inport
  Constant : Constant  Value=0
  Demux : Demux  Outputs=6
  Half-Bridge Converter : Subsystem
      settings: OpenFcn=elec.conv.unmask(gcb);
  Half-Bridge Converter1 : Subsystem
      settings: OpenFcn=elec.conv.unmask(gcb);
  Half-Bridge Converter2 : Subsystem
      settings: OpenFcn=elec.conv.unmask(gcb);
  Mux : Mux  Inputs=2
  Mux1 : Mux  Inputs=2
  Mux2 : Mux  Inputs=2
  Vdc+ : PMIOPort  Side=Left
  Vdc- : PMIOPort  Port=2  Side=Left
  Va : PMIOPort  Port=3  Side=Right
  Vb : PMIOPort  Port=4  Side=Right
  Vc : PMIOPort  Port=5  Side=Right
  wires:
  Mux2/1 -> Half-Bridge Converter2/1(" g ")
  Mux1/1 -> Half-Bridge Converter1/1(" g ")
  Mux/1 -> Half-Bridge Converter/1(" g ")
  Demux/6 -> Mux2/2
  Demux/5 -> Mux2/1
  Demux/3 -> Mux1/1
  Demux/4 -> Mux1/2
  Demux/2 -> Mux/2
  Demux/1 -> Mux/1
  Constant/1 -> Half-Bridge Converter/2(BL), Half-Bridge Converter1/2(BL), Half-Bridge Converter2/2(BL)
  g/1 -> Demux/1
  connections:
  Va/RConn1 -- Half-Bridge Converter/LConn1
  Vc/RConn1 -- Half-Bridge Converter2/LConn1
  Half-Bridge Converter1/LConn1 -- Vb/RConn1
  Half-Bridge Converter/RConn2 -- Half-Bridge Converter1/RConn2 -- Half-Bridge Converter2/RConn2 -- Vdc-/RConn1
  Vdc+/RConn1 -- Half-Bridge Converter1/RConn1 -- Half-Bridge Converter2/RConn1 -- Half-Bridge Converter/RConn1

== system PVAndBatteryIntegratedPlantForBlackStart/PV Inverter /L1 ==
  Three_PhaseSeriesRLCBran : ee_lib/Passive/RLC Assemblies/RLC (Three-Phase)  port_option=ee.enum.threePhasePort.expanded  component_structure=4  R=Rf Ohm  L=Lf H  C=Inf F  R_parasitic=1e-6 Ohm  G_parasitic=1e-6 1/Ohm  IL_specify=on  IL_priority=High  IL=[0, 0, 0] A  IL_nominal_specify=off  IL_nominal_value=1  IL_nominal_unit=A  VC_specify=on  VC_priority=High  VC=[0, 0, 0] V  VC_nominal_specify=off  VC_nominal_value=1  VC_nominal_unit=V
      settings: InternalSimscapePortConfiguration="{\"Bottom\":[],\"Left\":[{\"id\":\"a1\",\"label\":\"a1\",\"type\":\"foundation.electrical.electrical\"},{\"id\":\"b1\",\"label\":\"b1\",\"type\":\"foundation.electrical.electrical\"},{\"id\":\"c1\",\"label\":\"c1\",\"type\":\"foundation.electrical.electrical\"}],\"Right\":[{\"id\":\"a2\",\"label\":\"a2\",\"type\":\"foundation.electrical.electrical\"},{\"id\":\"b2\",\"label\":\"b2\",\"type\":\"foundation.electrical.electrical\"},{\"id\":\"c2\",\"label\":\"c2\",\"type\":\"foundation.electrical.electrical\"}],\"Top\":[]}"
  A : PMIOPort  Side=Left
  B : PMIOPort  Port=2  Side=Left
  C : PMIOPort  Port=3  Side=Left
  a : PMIOPort  Port=4  Side=Right
  b : PMIOPort  Port=5  Side=Right
  c : PMIOPort  Port=6  Side=Right
  connections:
  Three_PhaseSeriesRLCBran/RConn3 -- c/RConn1
  Three_PhaseSeriesRLCBran/RConn2 -- b/RConn1
  Three_PhaseSeriesRLCBran/RConn1 -- a/RConn1
  C/RConn1 -- Three_PhaseSeriesRLCBran/LConn3
  B/RConn1 -- Three_PhaseSeriesRLCBran/LConn2
  A/RConn1 -- Three_PhaseSeriesRLCBran/LConn1

== system PVAndBatteryIntegratedPlantForBlackStart/PV Inverter /Mosfet ==
  g : Inport
  Data Type Conversion : DataTypeConversion  OutDataTypeStr=double  SaturateOnIntegerOverflow=off  RndMeth=Floor
  MOSFET : ee_lib/Semiconductors & Converters/MOSFET (Ideal, Switching)  port_option=ee.enum.controlport.ps  Rds=Mosfet_class(0.01,100000,Inf,0.1,0).objParamMappingDerived.NewDerivedParam.Rds Ohm  Goff=Mosfet_class(0.01,100000,Inf,0.1,0).objParamMappingDerived.NewDerivedParam.Goff 1/Ohm  Vth=0.5 V  diode_param=2  diode_Vf=Mosfet_class(0.01,100000,Inf,0.1,0).objParamMappingDerived.NewDerivedParam.diode_Vf V  diode_Ron=Mosfet_class(0.01,100000,Inf,0.1,0).objParamMappingDerived.NewDerivedParam.diode_Ron Ohm  diode_Goff=Mosfet_class(0.01,100000,Inf,0.1,0).objParamMappingDerived.NewDerivedParam.diode_Goff 1/Ohm  diode_C=5e-8 F  diode_iRM=-235 A  diode_iF=300 A  diode_idot=-50 A/us  diode_trr_param=1  diode_trr_factor=3  diode_trr=15 us  diode_Qrr=1.5e+3 s*uA  ids_specify=off  ids_priority=None  ids=0 A  ids_nominal_specify=off  ids_nominal_value=1  ids_nominal_unit=A  vds_specify=off  vds_priority=None  vds=0 V  vds_nominal_specify=off  vds_nominal_value=1  vds_nominal_unit=V  vgs_specify=off  vgs_priority=None  vgs=0 V  vgs_nominal_specify=off  vgs_nominal_value=1  vgs_nominal_unit=V  thermal_loss_option=ee.enum.converters.thermalLossOption.constantvalues  Von_data=[0, 1.1, 1.3, 1.45, 1.75, 2.25, 2.7; 0, 1, 1.15, 1.35, 1.7, 2.35, 3] V  Tj=[298.15, 398.15] K  Iout_data=[0, 10, 50, 100, 200, 400, 600] A  Eon_data=[0, .29, 1.43, 2.86, 5.71, 13.14, 22.86; 0, .57, 2.63, 5.14, 10.29, 20.57, 30.29] * 1e-3 J  Eoff_data=[0, .21, 1.07, 2.14, 4.29, 9.86, 17.14; 0, .43, 1.97, 3.86, 7.71, 15.43, 22.71] * 1e-3 J  Eon_data_3D=[zeros(2, 5, 3)] J  Eoff_data_3D=[zeros(2, 5, 3)] J  Tj_loss=[298.15, 448.15] K  Iout_data_loss=[0, 10, 20, 30, 40] A  tabulateWithVds=false  Vds_loss=[0, 150, 300] V  Eon_scalar=22.86e-3 J  Eoff_scalar=17.14e-3 J  Voff=300 V  Iout_scalar=600 A  useCurrentFromPreviousCycle=false  useVoltageFromPreviousCycle=false  diodeModelType=ee.enum.converters.diodeModelType.pwl  diodeTableType=ee.enum.diode.tableType.IfMat  diode_ReverseIVType=ee.enum.diode.diodeReverseIV.constant  diode_IfMat=[.07, .12, .19, 1.75, 4.24, 7.32, 11.2; .16, .3, .72, 2.14, 4.02, 6.35, 9.12] A  diode_VfMat=[.9, 1.15, 1.25, 1.5, 1.75, 2.17, 2.6, 2.85; .58, .68, .75, 1.1, 1.38, 1.77, 2.27, 2.7] V  diode_TjVec=[25, 125] degC  diode_VfVec=[.5, .7, .9, 1.3, 1.7, 2.1, 2.5] V  diode_IfVec=[.1, .2, .5, 1, 2, 4, 7, 10] A  diode_IrMat=[1e-06, 2e-06, 5e-06, 1e-05, 2.5e-05, 5e-05, .0001; 2e-06, 5e-06, 1e-05, 4e-05, 8e-05, .0002, .0005] A  diode_VrMat=[10, 100, 200, 250, 300, 325, 350; 10, 70, 160, 220, 270, 300, 320] V  diode_VrVec=[10, 20, 40, 50, 70, 80, 100] V  diode_IrVec=[1e-06, 2e-06, 5e-06, 1e-05, 2e-05, 5e-05, .0001] A  diode_Vr=-600 V  diode_Ls=150 nH  diode_Erec=0.03 J  diode_rec_loss_model=ee.enum.diode.reverseRecoveryModel.fixed  diode_ErecVal=0 J  diode_scaleWithIandV=true  diode_ErecMat=zeros(2, 3) J  diode_TjrecVec=[298.15, 398.15] K  diode_IfrecVec=[.1, 1, 10] A  diode_IrecVal=10 A  diode_VrecVal=10 V  diode_tFilter=1 / 1000 / 100 s  separateThermalPortForDiode=false  thermal_network_parameterization=ee.enum.thermalNetworkTopology.external  Rth=[.03, .2] K/W  Rth_Cauer=[.03, .1, .2] K/W  Rth_Foster=[.03, .2] K/W  thermal_mass_parameterization=ee.enum.thermalNetwork.timeconstant  thermal_mass=[3, 25] J/K  thermal_mass_Cauer=[3, 10, 25] J/K  thermal_mass_Foster=[33, 50] J/K  thermal_time_constant=[.1, 5] s  thermal_time_constant_Cauer=[.1, 1, 5] s  thermal_time_constant_Foster=[1, 10] s  thermal_mass_initial_temperatures=[25, 25] degC  thermal_mass_initial_temperatures_Cauer=[25, 25, 25] degC  junction_thermal_mass=0.1 J/K  Tvec_initial_Foster=[25, 25, 25, 25] degC  RthDiode=[.03, .2] K/W  RthCauerDiode=[.03, .1, .2] K/W  RthFosterDiode=[.03, .2] K/W  thermalMassDiode=[3, 25] J/K  thermalMassCauerDiode=[3, 10, 25] J/K  thermalMassFosterDiode=[33, 50] J/K  thermalTauDiode=[.1, 5] s  thermalTauCauerDiode=[.1, 1, 5] s  thermalTauFosterDiode=[1, 10] s  thermalMassInitTempDiode=[25, 25] degC  thermalMassInitTempCauerDiode=[25, 25, 25] degC  junctionthermalMassDiode=0.1 J/K  TVecInitialFosterDiode=[25, 25, 25, 25] degC  no_thermal_network=0  mosfet_junction_temperature_specify=off  mosfet_junction_temperature_priority=None  mosfet_junction_temperature=25 degC  mosfet_junction_temperature_nominal_specify=off  mosfet_junction_temperature_nominal_value=1  mosfet_junction_temperature_nominal_unit=degC  diode_junction_temperature_specify=off  diode_junction_temperature_priority=None  diode_junction_temperature=25 degC  diode_junction_temperature_nominal_specify=off  diode_junction_temperature_nominal_value=1  diode_junction_temperature_nominal_unit=degC  Qj_specify=off  Qj_priority=None  Qj=0 W  Qj_nominal_specify=off  Qj_nominal_value=1  Qj_nominal_unit=W  accumulatedSwitchingLosses_specify=off  accumulatedSwitchingLosses_priority=None  accumulatedSwitchingLosses=0 J
  Simulink-PS Converter : nesl_utility/Simulink-PS Converter  PhysicalDomain=network_engine_domain  SubClassName=ps_input  LeftPortType=input  RightPortType=output  PseudoPeriodic=off  Frequencies=[]  NoiseDistribution=none  NoiseParameters=[]  Unit=1  AffineConversion=off  FilteringAndDerivatives=provide  SimscapeFilterOrder=1  InputFilterTimeConstant=0.001  UdotUserProvided=0
  D : PMIOPort  Side=Left
  S : PMIOPort  Port=2  Side=Right
  wires:
  g/1 -> Data Type Conversion/1
  Data Type Conversion/1 -> Simulink-PS Converter/1
  connections:
  S/RConn1 -- MOSFET/RConn2
  Simulink-PS Converter/RConn1 -- MOSFET/LConn1
  MOSFET/RConn1 -- D/RConn1
